simulink model "PID_Model"  (R2016a)
settings: Solver=ode15s  StartTime=0.0  StopTime=1500  MaxStep=1000  RelTol=1e-6
PostLoadFcn:
  | cd(fileparts(which(bdroot)))
undefined symbols (not defined in the file): Kd, Ki, Kp
settings Model: ModifiedByFormat=Mars  ModifiedHistory=Modified by YiXiuKeJi; Taobao is : https://shop197632247.taobao.com  Creator=一休科技  LastModifiedBy=Mars
settings DataIOCC: LimitDataPoints=on  SaveFormat=Array  SignalLoggingSaveFormat=ModelDataLogs  SignalLoggingName=sigsOut
settings OptimizationCC: ExpressionDepthLimit=2147483647  InitFltsAndDblsToZero=on
settings DebuggingCC: SaveWithParameterizedLinksMsg=none  UnderspecifiedInitializationDetection=Classic  MergeDetectMultiDrivingBlocksExec=none  SignalResolutionControl=TryResolveAllWithWarning  MultiTaskDSMMsg=warning  MultiTaskCondExecSysMsg=none  FcnCallInpInsideContextMsg=EnableAllAsWarning  StateNameClashWarn=warning
settings HardwareCC: ProdBitPerPointer=32  ProdLargestAtomicFloat=None  ProdIntDivRoundTo=Undefined  ProdEndianess=Unspecified  ProdWordSize=32  ProdHWDeviceType=32-bit Generic  TargetUnknown=on
settings ModelReferenceCC: PropagateSignalLabelsOutOfModel=off
settings GRTTargetCC: TargetFcnLib=ansi_tfl_tmw.mat  CombineOutputUpdateFcns=off  GRTInterface=on
settings ConfigComp: CovSFcnEnable=off

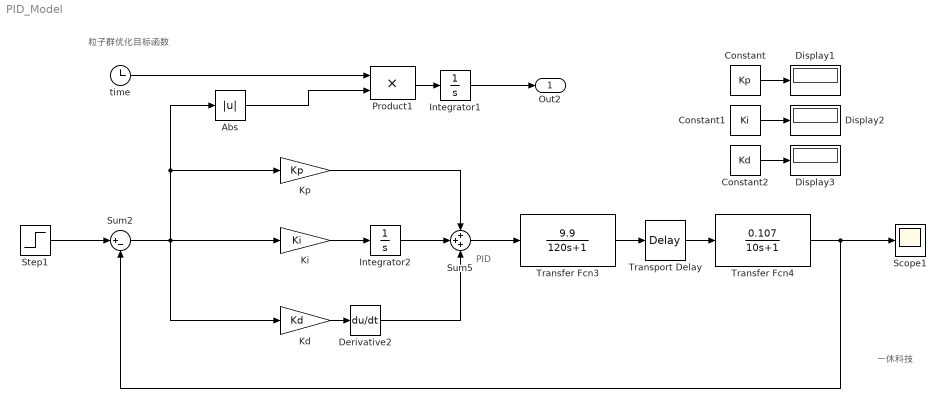
== system PID_Model ==
  note: PID
  note: 粒子群优化目标函数
  note: 一休科技
  Abs : Abs  ZeroCross=off  SaturateOnIntegerOverflow=on
  Constant : Constant  Value=Kp
  Constant1 : Constant  Value=Ki
  Constant2 : Constant  Value=Kd
  Derivative2 : Derivative
  Display1 : Display
  Display2 : Display
  Display3 : Display
  Integrator1 : Integrator
  Integrator2 : Integrator
  Kd : Gain  Gain=Kd
  Ki : Gain  Gain=Ki
  Kp : Gain  Gain=Kp
  Product1 : Product  SaturateOnIntegerOverflow=on  OutDataTypeStr=Inherit: Same as first input
  Scope1 : Scope
  Step1 : Step  Time=0  After=100  SampleTime=0
  Sum2 : Sum  Inputs=|+-  SaturateOnIntegerOverflow=on
  Sum5 : Sum  Inputs=+++
  Transfer Fcn3 : TransferFcn  Numerator=[9.9 ]  Denominator=[120 1]
  Transfer Fcn4 : TransferFcn  Numerator=[0.107]  Denominator=[10 1]
  Transport Delay : TransportDelay  DelayTime=80
  time : Clock
  Out2 : Outport
  wires:
  time/1 -> Product1/1
  Integrator1/1 -> Out2/1
  Product1/1 -> Integrator1/1
  Derivative2/1 -> Sum5/3
  Integrator2/1 -> Sum5/2
  Sum2/1 -> Kd/1, Kp/1, Abs/1, Ki/1
  Sum5/1 -> Transfer Fcn3/1
  Ki/1 -> Integrator2/1
  Transfer Fcn4/1 -> Scope1/1, Sum2/2
  Step1/1 -> Sum2/1
  Transfer Fcn3/1 -> Transport Delay/1
  Transport Delay/1 -> Transfer Fcn4/1
  Kd/1 -> Derivative2/1
  Kp/1 -> Sum5/1
  Constant/1 -> Display1/1
  Constant1/1 -> Display2/1
  Constant2/1 -> Display3/1
  Abs/1 -> Product1/2
